simulink model "npc_controller"  (R2022a)
settings: Solver=FixedStepDiscrete  StartTime=0.0  StopTime=20  RelTol=1e-3  EnableMultiTasking=on
undefined symbols (not defined in the file): CAN_O_INT, CANA_BASE, Down, GPTRIP1SEL, GPTRIP2SEL, GPTRIP3SEL, Tsw, TZ1, TZ2, TZ3, Up
libraries: simulink x147, hdlsllib x90, c2802xlib x34, c2837xDlib x20, c280xlib x12, canmsglib x9, c2838xlib x8, idelinklib_common x3, c2806xlib x2, slpidlib x2, c28004xlib x2, c281xlib x2
(part 42 of 42)

== stateflow chart npc_controller/CONTROL/STATE-MACHINE/CPU_CONTROL_750_A2_precharge_pfc_ok2_OL SS1/detectUvpOvp/UVP ==
  (default) -> (junction 26)
  (junction 26) -> (junction 19) [order 1] : [Vpk2 < 536] %170Vacrms
  (junction 26) -> (junction 22) [order 2]
  (junction 19) -> (junction 23) : {
      | tfv_v_Uvp = 1; %set the UVP flag
      | }
  (junction 22) -> (junction 20) [order 1] : [Vpk2 > 568] %180Vacrms
  (junction 22) -> (junction 28) [order 2]
  (junction 20) -> (junction 18) : {
      | tfv_v_Uvp = 0;
      | }
  (junction 28) -> (junction 18)
  (junction 18) -> (junction 23)
  data: Vpk2 input single; tfv_v_Uvp output double

== stateflow chart npc_controller/CONTROL/STATE-MACHINE/CPU_CONTROL_750_A2_precharge_pfc_ok2_OL SS2 ==
  state configGrid(grid_config,   sinlgeph_config) [function] [commented out]
  state ClrCmpssTz [function] [commented out]
  state configFutEn [function]
  state disCmpssTz [function] [commented out]
  state configFutDis [function]
  state readCmpssOcp [function]
  state theta = updatePll3p(van, vbn, vcn) [function] [commented out]
  state calib_ok = updateCalib(cnt_calib, van, vbn, vcn, ia, ib, ic) [function]
  state disablePwm [function]
  state tfv_v_UvpOvp = detectUvpOvp(Vpk) [function]
  state phx_en = detectZCPhA(vxn) [function]
  state phx_en = detectZCPhB(vxn) [function]
  state phx_en = detectZCPhC(vxn) [function]
  state vx_seq = updateSequencePhA(vxn, ix) [function]
  state vx_seq = updateSequencePhB(vxn, ix) [function]
  state vx_seq = updateSequencePhC(vxn, ix) [function]
  (default) -> (junction 597)
  (junction 598) -> (junction 531) [order 1] : [calib_ok]
      | {tfv_v_UvpOvp = 0;//detectUvpOvp(Vpk);
      | readCmpssOcp();
      | }
  (junction 597) -> (junction 598) [order 1] : [start_cnt>1]%63333]//50cycles
  (junction 531) -> (junction 14)
  (junction 597) -> (junction 601) [order 2] : {
      | start_cnt++;
      | //disCmpssTz();
      | }
      | //exit
  (junction 598) -> (junction 539) [order 2] : {
      | calib_ok = updateCalib(cnt_calib, van, vbn, vcn, ia, ib, ic);
      | state = 0;
      | }
      | //exit
  (junction 14) -> (junction 542) [order 2]
  (junction 542) -> (junction 504) [order 2]
  (junction 504) -> (junction 506) [order 1] : [fut_en]
  (junction 14) -> (junction 128) [order 1] : /*fault latch*/
      | [tfv_va || tfv_vb || tfv_vc || tfv_iphasea || tfv_iphaseb || tfv_iphasec || tfv_vbulk || tfv_vmid /*|| tfv_vtop*/ || tfv_vaux || tz_ocp || tz_ovp || tz_cmpssocp || fault]
      | {
      | fault = true;
      | state = 1;
      | }
      | //turn OFF
  (junction 542) -> (junction 501) [order 1]
  (junction 504) -> (junction 512) [order 2]
  (junction 506) -> (junction 508) : {
      | configFutDis();
      | fut_en = false;
      | }
  (junction 508) -> (junction 512)
  (junction 501) -> (junction 490) : [fut_en_req]
  (junction 512) -> (junction 739)
  (junction 739) -> (junction 742) [commented out]
  (junction 490) -> (junction 492) [order 1] : [!fut_en]
  (junction 739) -> (junction 745) [order 2]
  (junction 742) -> (junction 735) [commented out] : [control_en]
  (junction 492) -> (junction 498) : {
      | configFutEn();
      | fut_en = true;
      | }
  (junction 490) -> (junction 494) [order 2]
  (junction 745) -> (junction 762) : {state = 7;}
      | //turn OFF
  (junction 739) -> (junction 734) [order 1] : [!tfv_v_UvpOvp]//check ac_ok at start
  (junction 494) -> (junction 498)
  (junction 735) -> (junction 734) [commented out]
  (junction 498) -> (junction 520) : {state = 2;}
  (junction 734) -> (junction 721)
  (junction 676) -> (junction 679) [order 1] : [control_en]
  (junction 721) -> (junction 712) [order 1] : [!pfc_en]
      | {state = 6;}
      | //turn OFF
      | //relay OFF
  (junction 721) -> (junction 778) [order 2]
  (junction 778) -> (junction 676) [order 1] : [delay_cnt > 100]//2666]
  (junction 679) -> (junction 678)
  (junction 778) -> (junction 780) [order 2] : {delay_cnt++;}
      | //exit
  (junction 676) -> (junction 346) [order 2]
  (junction 712) -> (junction 713)
  (junction 346) -> (junction 626) [order 1] : [(1.9797*2*Vpk-vbulk) < 50]
  (junction 346) -> (junction 558) [order 2]
  (junction 626) -> (junction 658) : {relay_ctrl = 1; //pre-charge relay ON
      | }
  (junction 658) -> (junction 678)
  (junction 678) -> (junction 622) [order 1] : [1]//relay_ctrl]
  (junction 558) -> (junction 658)
  (junction 622) -> (junction 624) [order 1] : [relay_cnt > 100]//3300] //PWM ON with 40ms delay
  (junction 624) -> (junction 754) [order 1] : [control_en]
  (junction 678) -> (junction 707) [order 2] : //exit
  (junction 622) -> (junction 623) [order 2] : {relay_cnt++;}
      | //exit
  (junction 624) -> (junction 699) [order 2]
  (junction 754) -> (junction 684)
  (junction 699) -> (junction 698) [order 1] : [vbulk > 2385] //540V
  (junction 699) -> (junction 692) [order 2]
  (junction 698) -> (junction 696) : {
      | control_en = 1; //PWM ON
      | ref = vbulk;
      | //enDigCmpMode();
      | //enCmpssTz();
      | }
  (junction 692) -> (junction 689) [order 1] : [vbulk < 2209] //500V
  (junction 692) -> (junction 691) [order 2]
  (junction 689) -> (junction 695) : {
      | control_en = false;
      | }
  (junction 684) -> (junction 114) [order 1] : [control_en]
  (junction 114) -> (junction 266) [order 1] : [vbulk > 5711] //840V
  (junction 696) -> (junction 684)
  (junction 691) -> (junction 695)
  (junction 695) -> (junction 696)
  (junction 684) -> (junction 665) [order 2] : //exit
  (junction 114) -> (junction 263) [order 2]
  (junction 266) -> (junction 273) : {
      | eoss = false;
      | burst_en = true;
      | }
  (junction 263) -> (junction 264) [order 1] : [vbulk < 3314] //750V
  (junction 263) -> (junction 267) [order 2]
  (junction 264) -> (junction 270) : {burst_en = false;}
  (junction 267) -> (junction 270)
  (junction 270) -> (junction 273)
  (junction 273) -> (junction 276) [order 1] : [burst_en]
  (junction 273) -> (junction 254) [order 2]
  (junction 276) -> (junction 327) : {
      | disablePwm();
      | va_seq = uint8(0); //forced zero
      | vb_seq = uint8(0);
      | vc_seq = uint8(0);
      | pha_en = false;
      | phb_en = false;
      | phc_en = false;
      | state = 5;
      | }
  (junction 254) -> (junction 256) [order 1] : [eoss]
      | //{tfv_v_UvpOvp = detectUvpOvp(Vpk)}
  (junction 256) -> (junction 648) [order 1] : [eoss_cnt > 6667]//5cycles delay after SS for PFC_OK
  (junction 254) -> (junction 97) [order 2]
  (junction 256) -> (junction 101) [order 2] : {
      | eoss_cnt++;
      | pfc_ok = 0;
      | }
  (junction 648) -> (junction 647) : {pfc_ok = 1;
      | /*eoss_cnt = 13100;*/}
  (junction 580) -> (junction 581) [commented out] : [(grid_config_req != grid_config) || (singleph_config_req != singleph_config)]
  (junction 97) -> (junction 93) [order 1] : [ref < 3314]%(single(883)-vbulk) > single(50)] //11V ripple
  (junction 580) -> (junction 583) [commented out]
  (junction 581) -> (junction 582) [commented out] : {
      | configGrid(grid_config,   singleph_config);
      | grid_config = grid_config_req;
      | singleph_config = singleph_config_req;
      | }
  (junction 97) -> (junction 110) [order 2]
  (junction 93) -> (junction 109) : {ref = ref + single(50);
      | eoss = false;}
  (junction 110) -> (junction 96) [commented out] : [(single(883)-vbulk) < single(-50)]
  (junction 110) -> (junction 94) : {ref = single(3314); //750V
      | eoss = true;}
  (junction 96) -> (junction 108) [commented out] : {ref = vbulk - single(1);
      | eoss = false;}
  (junction 101) -> (junction 647)
  (junction 647) -> (junction 352) [order 1] : [pha_en]
  (junction 109) -> (junction 101)
  (junction 582) -> (junction 583) [commented out]
  (junction 94) -> (junction 108)
  (junction 108) -> (junction 109)
  (junction 647) -> (junction 356) [order 2] : {
      | va_seq = uint8(0);
      | pha_en = detectZCPhA(van);
      | }
  (junction 352) -> (junction 354) : {va_seq = updateSequencePhA(van, ia);}
  (junction 583) -> (junction 133) [commented out]
  (junction 356) -> (junction 354)
  (junction 354) -> (junction 362) [order 1] : [phb_en]
  (junction 354) -> (junction 365) [order 2] : {
      | vb_seq = uint8(0);
      | phb_en = detectZCPhB(vbn);
      | }
  (junction 362) -> (junction 366) : {vb_seq = updateSequencePhB(vbn, ib);}
  (junction 365) -> (junction 366)
  (junction 366) -> (junction 367) [order 1] : [phc_en]
  (junction 366) -> (junction 370) [order 2] : {
      | vc_seq = uint8(0);
      | phc_en = detectZCPhC(vcn);
      | }
  (junction 367) -> (junction 372) : {vc_seq = updateSequencePhC(vcn, ic);}
  (junction 370) -> (junction 372)
  (junction 372) -> (junction 299) : {state = 4;}
  (junction 757) -> (junction 635) [order 1] : [!pfc_en || tfv_v_UvpOvp]
  (junction 635) -> (junction 299) [order 1] : [relayOff_cnt>2600] //40ms delay to turn-OFF pre-charge relay
      | {
      | relay_ctrl = 0; //pre-charge relay OFF
      | relayOff_cnt = 0;
      | relay_cnt = 0;
      | eoss_cnt = 0;
      | delay_cnt = 0;
      | }
  (junction 128) -> (junction 762) : //{calib_ok = false;} //calib_ok resets at fault or CAN command
  (junction 762) -> (junction 713)
  (junction 713) -> (junction 133)
  (junction 299) -> (junction 327)
  (junction 133) -> (junction 757) : {
      | disablePwm();
      | eoss = false;
      | //disDigCmpMode();
      | pha_en = false;
      | phb_en = false;
      | phc_en = false;
      | ref = vbulk;
      | %state = 3;
      | pfc_ok = 0;
      | control_en = false;
      | }
  (junction 635) -> (junction 637) [order 2] : {relayOff_cnt++;}
  (junction 632) -> (junction 299)
  (junction 327) -> (junction 533)
  (junction 757) -> (junction 759) [order 2]
  (junction 637) -> (junction 632)
  (junction 539) -> (junction 520)
  (junction 520) -> (junction 731)
  (junction 731) -> (junction 780)
  (junction 780) -> (junction 707)
  (junction 707) -> (junction 623)
  (junction 623) -> (junction 665)
  (junction 665) -> (junction 759)
  (junction 759) -> (junction 533)
  (junction 601) -> (junction 539)
  data: grid_config function_input double size=1; sinlgeph_config function_input double size=1; van function_input double size=1; vbn function_input double size=1; vcn function_input double size=1; theta function_output double size=1; calib_ok function_output; cnt_calib function_input uint16 size=1; van function_input single size=1; vbn function_input single size=1; vcn function_input single size=1; ia function_input single size=1; ib function_input single size=1; ic function_input single size=1; Vpk function_input; tfv_v_UvpOvp function_output; vxn function_input; phx_en function_output; vxn function_input; phx_en function_output; vxn function_input; phx_en function_output; vxn function_input; vx_seq function_output; ix function_input; vxn function_input; vx_seq function_output; ix function_input; vxn function_input; vx_seq function_output; ix function_input; state output uint16 =0; calib_ok output boolean =false; van input single; vbn input single; vcn input single; ia input single; ib input single; ic input single; tfv_vbulk data_store_memory; tfv_va data_store_memory; tfv_vmid data_store_memory; tfv_vb data_store_memory; tfv_vc data_store_memory; tfv_iphasea data_store_memory; tfv_iphaseb data_store_memory; tfv_iphasec data_store_memory; tfv_vtop data_store_memory; control_en output boolean =false; burst_en output boolean =false; eoss output boolean =false; ref output single =0; va_seq output uint8 =false; vb_seq output uint8 =false; vc_seq output uint8 =false; vbulk input single; fault local boolean =false; cnt_calib data_store_memory =0; theta data_store_memory =0; fut_en_req input uint8; fut_en local boolean =false; tfv_vaux data_store_memory; tz_ocp data_store_memory; tz_ovp data_store_memory; cnt_200ms local uint16 =0; pha_en output boolean =false; phb_en output boolean =false; phc_en output boolean =false; grid_config_req input uint8; singleph_config_req input uint8; grid_config local uint8 =0; singleph_config local uint8 =0; start_cnt local double; Vpk input single; relayOff_cnt local double; relay_cnt local double; pfc_ok output boolean; eoss_cnt local double; relay_ctrl output boolean; pfc_en input; tfv_v_UvpOvp output boolean; delay_cnt local double; tz_cmpssocp data_store_memory

== stateflow chart npc_controller/CONTROL/STATE-MACHINE/CPU_CONTROL_750_A2_precharge_pfc_ok2_OL SS2/detectUvpOvp/OVP ==
  (default) -> (junction 5)
  (junction 5) -> (junction 4) [order 1] : [Vpk1 > 773] %245Vacrms
  (junction 5) -> (junction 7) [order 2]
  (junction 4) -> (junction 6) : {
      | tfv_v_Ovp = 1; %set the OVP flag
      | }
  (junction 7) -> (junction 2) [order 1] : [Vpk1 < 741] %235Vacrms
  (junction 7) -> (junction 1) [order 2]
  (junction 2) -> (junction 3) : {
      | tfv_v_Ovp = 0;
      | }
  (junction 1) -> (junction 3)
  (junction 3) -> (junction 6)
  data: Vpk1 input single; tfv_v_Ovp output double

== stateflow chart npc_controller/CONTROL/STATE-MACHINE/CPU_CONTROL_750_A2_precharge_pfc_ok2_OL SS2/detectUvpOvp/UVP ==
  (default) -> (junction 26)
  (junction 26) -> (junction 19) [order 1] : [Vpk2 < 536] %170Vacrms
  (junction 26) -> (junction 22) [order 2]
  (junction 19) -> (junction 23) : {
      | tfv_v_Uvp = 1; %set the UVP flag
      | }
  (junction 22) -> (junction 20) [order 1] : [Vpk2 > 568] %180Vacrms
  (junction 22) -> (junction 28) [order 2]
  (junction 20) -> (junction 18) : {
      | tfv_v_Uvp = 0;
      | }
  (junction 28) -> (junction 18)
  (junction 18) -> (junction 23)
  data: Vpk2 input single; tfv_v_Uvp output double

== stateflow chart npc_controller/CONTROL/SVPWM/SVPWM_with_bal ==
  state [Tx,Ty,Tz] = calcDwellingTimes(Tsw,vref_fict_mag_alpha,vref_fict_mag_beta,vx_fict_mag_alpha,vx_fict_mag_beta,vy_fict_mag_alpha,vy_fict_mag_beta) [function]
  state [r_seq, s_seq, t_seq]=detSeq(subsector) [function]
  state [r_seq, s_seq, t_seq]=detSeqFixedSmallVector(subsector) [function] [commented out]
  state [cmp_r, cmp_s, cmp_t] = calcCmp(r_seq, s_seq, t_seq, Tx, Ty, Tz) [function] [commented out]
  state [cmp_r, cmp_s, cmp_t] = calcCmpWithBal(r_seq, s_seq, t_seq, Tx, Ty, Tz) [function]
  (default) -> (junction 4)
  (junction 4) -> (junction 6) [order 1] : [vref_mag_alpha >= 0]
  (junction 6) -> (junction 12) [order 1] : [vref_mag_beta >= 0]
  (junction 12) -> (junction 14) [order 1] : [vref_mag_beta > (vref_mag_alpha*tan(3.14/6))]
  (junction 4) -> (junction 8) [order 2]
  (junction 6) -> (junction 23) [order 2]
  (junction 12) -> (junction 19) [order 2] : {main_sector = 1;}
  (junction 14) -> (junction 16) : {main_sector = 2;}
  (junction 19) -> (junction 16)
  (junction 16) -> (junction 54)
  (junction 23) -> (junction 25) [order 1] : [vref_mag_beta < (-vref_mag_alpha*tan(3.14/6))]
  (junction 23) -> (junction 29) [order 2] : {main_sector = 1;}
  (junction 25) -> (junction 27) : {main_sector = 6;}
  (junction 29) -> (junction 27)
  (junction 27) -> (junction 54)
  (junction 54) -> (junction 52)
  (junction 32) -> (junction 39) [order 1] : [vref_mag_beta > (abs(vref_mag_alpha)*tan(3.14/6))]
  (junction 8) -> (junction 32) [order 1] : [vref_mag_beta >= 0]
  (junction 39) -> (junction 40) : {main_sector = 3;}
  (junction 8) -> (junction 35) [order 2]
  (junction 32) -> (junction 41) [order 2] : {main_sector = 4;}
  (junction 41) -> (junction 40)
  (junction 40) -> (junction 52)
  (junction 52) -> (junction 21)
  (junction 35) -> (junction 44) [order 1] : [vref_mag_beta < (vref_mag_alpha*tan(3.14/6))]
  (junction 35) -> (junction 46) [order 2] : {main_sector = 4;}
  (junction 44) -> (junction 48) : {main_sector = 5;}
  (junction 46) -> (junction 48)
  (junction 48) -> (junction 21)
  (junction 21) -> (junction 63)
  (junction 63) -> (junction 64) [order 1] : [main_sector == 1]
  (junction 63) -> (junction 65) [order 2]
  (junction 64) -> (junction 86) : {
      | mapv_mag_alpha = 0.3333;
      | mapv_mag_beta = 0;
      | }
  (junction 65) -> (junction 69) [order 1] : [main_sector == 2]
  (junction 65) -> (junction 67) [order 2]
  (junction 69) -> (junction 72) : {
      | mapv_mag_alpha = 0.1667;
      | mapv_mag_beta = 0.2887;
      | }
  (junction 67) -> (junction 68) [order 1] : [main_sector == 3]
  (junction 67) -> (junction 58) [order 2]
  (junction 68) -> (junction 95) : {
      | mapv_mag_alpha = -0.1667;
      | mapv_mag_beta = 0.2887;
      | }
  (junction 58) -> (junction 66) [order 1] : [main_sector == 4]
  (junction 58) -> (junction 59) [order 2]
  (junction 66) -> (junction 93) : {
      | mapv_mag_alpha = -0.3333;
      | mapv_mag_beta = 0;
      | }
  (junction 59) -> (junction 60) [order 1] : [main_sector == 5]
  (junction 59) -> (junction 61) [order 2]
  (junction 60) -> (junction 91) : {
      | mapv_mag_alpha = -0.1667;
      | mapv_mag_beta = -0.2887;
      | }
  (junction 61) -> (junction 62) [order 1] : [main_sector == 6]
  (junction 61) -> (junction 83) [order 2]
  (junction 62) -> (junction 90) : {
      | mapv_mag_alpha = 0.1667;
      | mapv_mag_beta = -0.2887;
      | }
  (junction 83) -> (junction 90)
  (junction 90) -> (junction 91)
  (junction 91) -> (junction 93)
  (junction 93) -> (junction 95)
  (junction 95) -> (junction 72)
  (junction 72) -> (junction 86)
  (junction 86) -> (junction 145) : {
      | vref_fict_mag_alpha = vref_mag_alpha - mapv_mag_alpha;
      | vref_fict_mag_beta = vref_mag_beta - mapv_mag_beta;
      | }
  (junction 145) -> (junction 146) [order 1] : [vref_fict_mag_alpha >= 0]
  (junction 146) -> (junction 147) [order 1] : [vref_fict_mag_beta >= 0]
  (junction 147) -> (junction 148) [order 1] : [vref_fict_mag_beta > (vref_fict_mag_alpha*tan(3.14/3))]
  (junction 145) -> (junction 158) [order 2]
  (junction 146) -> (junction 149) [order 2]
  (junction 147) -> (junction 150) [order 2] : {subsector = 1;}
  (junction 148) -> (junction 151) : {subsector = 2;}
  (junction 150) -> (junction 151)
  (junction 151) -> (junction 159)
  (junction 149) -> (junction 152) [order 1] : [vref_fict_mag_beta < (-vref_fict_mag_alpha*tan(3.14/3))]
  (junction 149) -> (junction 153) [order 2] : {subsector = 6;}
  (junction 152) -> (junction 154) : {subsector = 5;}
  (junction 153) -> (junction 154)
  (junction 154) -> (junction 159)
  (junction 159) -> (junction 109)
  (junction 156) -> (junction 155) [order 1] : [vref_fict_mag_beta > (abs(vref_fict_mag_alpha)*tan(3.14/3))]
  (junction 158) -> (junction 156) [order 1] : [vref_fict_mag_beta >= 0]
  (junction 155) -> (junction 122) : {subsector = 2;}
  (junction 158) -> (junction 126) [order 2]
  (junction 156) -> (junction 157) [order 2] : {subsector = 3;}
  (junction 157) -> (junction 122)
  (junction 122) -> (junction 109)
  (junction 109) -> (junction 128)
  (junction 126) -> (junction 127) [order 1] : [vref_fict_mag_beta < (vref_fict_mag_alpha*tan(3.14/3))]
  (junction 126) -> (junction 129) [order 2] : {subsector = 4;}
  (junction 127) -> (junction 130) : {subsector = 5;}
  (junction 129) -> (junction 130)
  (junction 130) -> (junction 128)
  (junction 128) -> (junction 182)
  (junction 182) -> (junction 162) [order 1] : [subsector == 1]
  (junction 182) -> (junction 163) [order 2]
  (junction 162) -> (junction 179) : {
      | vx_fict_mag_alpha = 0.3333;
      | vx_fict_mag_beta = 0;
      | vy_fict_mag_alpha = 0.1667;
      | vy_fict_mag_beta = 0.2887;
      | }
  (junction 163) -> (junction 164) [order 1] : [subsector == 2]
  (junction 163) -> (junction 177) [order 2]
  (junction 164) -> (junction 178) : {
      | vx_fict_mag_alpha = 0.1667;
      | vx_fict_mag_beta = 0.2887;
      | vy_fict_mag_alpha = -0.1667;
      | vy_fict_mag_beta = 0.2887;
      | }
  (junction 177) -> (junction 167) [order 1] : [subsector == 3]
  (junction 177) -> (junction 174) [order 2]
  (junction 167) -> (junction 172) : {
      | vx_fict_mag_alpha = -0.1667;
      | vx_fict_mag_beta = 0.2887;
      | vy_fict_mag_alpha = -0.3333;
      | vy_fict_mag_beta = 0;
      | }
  (junction 174) -> (junction 173) [order 1] : [subsector == 4]
  (junction 174) -> (junction 175) [order 2]
  (junction 173) -> (junction 170) : {
      | vx_fict_mag_alpha = -0.3333;
      | vx_fict_mag_beta = 0;
      | vy_fict_mag_alpha = -0.1667;
      | vy_fict_mag_beta = -0.2887;
      | }
  (junction 175) -> (junction 165) [order 1] : [subsector == 5]
  (junction 175) -> (junction 166) [order 2]
  (junction 165) -> (junction 176) : {
      | vx_fict_mag_alpha = -0.1667;
      | vx_fict_mag_beta = -0.2887;
      | vy_fict_mag_alpha = 0.1667;
      | vy_fict_mag_beta = -0.2887;
      | }
  (junction 166) -> (junction 171) [order 1] : [subsector == 6]
  (junction 166) -> (junction 168) [order 2]
  (junction 171) -> (junction 169) : {
      | vx_fict_mag_alpha = 0.1667;
      | vx_fict_mag_beta = -0.2887;
      | vy_fict_mag_alpha = 0.3333;
      | vy_fict_mag_beta = 0;
      | }
  (junction 168) -> (junction 169)
  (junction 169) -> (junction 176)
  (junction 176) -> (junction 170)
  (junction 170) -> (junction 172)
  (junction 172) -> (junction 178)
  (junction 178) -> (junction 179)
  (junction 179) -> (junction 232) : {
      | [Tx, Ty, Tz] = calcDwellingTimes(Tsw, vref_fict_mag_alpha, vref_fict_mag_beta, vx_fict_mag_alpha, vx_fict_mag_beta, vy_fict_mag_alpha, vy_fict_mag_beta);
      | }
  (junction 232) -> (junction 247) : {
      | [r_seq, s_seq, t_seq]=detSeq(subsector);
      | }
  (junction 247) -> (junction 334) : {[cmp_r, cmp_s, cmp_t] = calcCmpWithBal(r_seq, s_seq, t_seq, Tx, Ty, Tz);}
  (junction 334) -> (junction 262)
  (junction 262) -> (junction 253) [order 1] : [main_sector == 1]
  (junction 262) -> (junction 258) [order 2]
  (junction 253) -> (junction 283) : {
      | r_p = cmp_r+midpt_bal_coef;
      | r_n = 0;
      | s_p = 0;
      | s_n = -cmp_s+1;
      | t_p = 0;
      | t_n = -cmp_t+1;
      | }
  (junction 258) -> (junction 254) [order 1] : [main_sector == 2]
  (junction 258) -> (junction 255) [order 2]
  (junction 254) -> (junction 276) : {
      | r_p = cmp_r+midpt_bal_coef;
      | r_n = 0;
      | s_p = cmp_s+midpt_bal_coef;
      | s_n = 0;
      | t_p = 0;
      | t_n = -cmp_t+1;
      | }
  (junction 255) -> (junction 250) [order 1] : [main_sector == 3]
  (junction 255) -> (junction 256) [order 2]
  (junction 250) -> (junction 266) : {
      | r_p = 0;
      | r_n = -cmp_r+1;
      | s_p = cmp_s+midpt_bal_coef;
      | s_n = 0;
      | t_p = 0;
      | t_n = -cmp_t+1;
      | }
  (junction 256) -> (junction 257) [order 1] : [main_sector == 4]
  (junction 256) -> (junction 261) [order 2]
  (junction 257) -> (junction 265) : {
      | r_p = 0;
      | r_n = -cmp_r+1;
      | s_p = cmp_s+midpt_bal_coef;
      | s_n = 0;
      | t_p = cmp_t+midpt_bal_coef;
      | t_n = 0;
      | }
  (junction 261) -> (junction 251) [order 1] : [main_sector == 5]
  (junction 261) -> (junction 259) [order 2]
  (junction 251) -> (junction 264) : {
      | r_p = 0;
      | r_n = -cmp_r+1;
      | s_p = 0;
      | s_n = -cmp_s+1;
      | t_p = cmp_t+midpt_bal_coef;
      | t_n = 0;
      | }
  (junction 259) -> (junction 260) [order 1] : [main_sector == 6]
  (junction 259) -> (junction 252) [order 2]
  (junction 260) -> (junction 263) : {
      | r_p = cmp_r+midpt_bal_coef;
      | r_n = 0;
      | s_p = 0;
      | s_n = -cmp_s+1;
      | t_p = cmp_t+midpt_bal_coef;
      | t_n = 0;
      | }
  (junction 252) -> (junction 263)
  (junction 263) -> (junction 264)
  (junction 264) -> (junction 265)
  (junction 265) -> (junction 266)
  (junction 266) -> (junction 276)
  (junction 276) -> (junction 283)
  (junction 283) -> (junction 316) : {
      | debug_a = main_sector;
      | debug_b = subsector;
      | debug_c = cmp_r;
      | }
  data: Tsw function_input double size=1; vref_fict_mag_alpha function_input double size=1; vref_fict_mag_beta function_input double size=1; Tx function_output; Ty function_output; Tz function_output; vx_fict_mag_alpha function_input double size=1; vx_fict_mag_beta function_input double size=1; vy_fict_mag_alpha function_input double size=1; vy_fict_mag_beta function_input double size=1; subsector function_input double size=1; r_seq function_output; s_seq function_output; t_seq function_output; subsector function_input double size=1; r_seq function_output double size=1; s_seq function_output double size=1; t_seq function_output double size=1; r_seq function_input double size=1; cmp_r function_output double size=1; cmp_s function_output double size=1; cmp_t function_output double size=1; s_seq function_input double size=1; t_seq function_input double size=1; Tx function_input double size=1; Ty function_input double size=1; Tz function_input double size=1; r_seq function_input double size=4; cmp_r function_output; cmp_s function_output; cmp_t function_output; s_seq function_input double size=4; t_seq function_input double size=4; Tx function_input double size=1; Ty function_input double size=1; Tz function_input double size=1; r_p output double; r_n output double; vref_mag_alpha input double; vref_mag_beta input double; mapv_mag_alpha local double; mapv_mag_beta local double; vref_fict_mag_alpha local double; vref_fict_mag_beta local double; subsector local double; main_sector local double; vx_fict_mag_alpha local double; vx_fict_mag_beta local double; vy_fict_mag_alpha local double; vy_fict_mag_beta local double; midpt_bal_coef input double; Tx local double; Ty local double; Tz local double; s_p output double; s_n output double; t_p output double; t_n output double; cmp_r local double; cmp_s local double; cmp_t local double; r_seq local double size=4; s_seq local double size=4; t_seq local double size=4; debug_a output double; debug_b output double; debug_c output double; Tsw input double

== stateflow chart npc_controller/CONTROL/SVPWM/SVPWM2 ==
  state [Tx,Ty,Tz] = calcDwellingTimes(Tsw,vref_fict_mag_alpha,vref_fict_mag_beta,vx_fict_mag_alpha,vx_fict_mag_beta,vy_fict_mag_alpha,vy_fict_mag_beta) [function]
  state [r_seq, s_seq, t_seq]=detSeq(subsector) [function]
  state [cmp_r,cmp_s,cmp_t] = calcCmpBal(r_seq,s_seq,t_seq,Tx,Ty,Tz,vbal_coef) [function]
  (default) -> (junction 4)
  (junction 4) -> (junction 6) [order 1] : [vref_mag_alpha >= 0]
  (junction 6) -> (junction 12) [order 1] : [vref_mag_beta >= 0]
  (junction 12) -> (junction 14) [order 1] : [vref_mag_beta > (vref_mag_alpha*0.5774)]
  (junction 4) -> (junction 8) [order 2]
  (junction 6) -> (junction 23) [order 2]
  (junction 12) -> (junction 19) [order 2] : {main_sector = 1;}
  (junction 14) -> (junction 16) : {main_sector = 2;}
  (junction 19) -> (junction 16)
  (junction 16) -> (junction 54)
  (junction 23) -> (junction 25) [order 1] : [vref_mag_beta < (-vref_mag_alpha*0.5774)]
  (junction 23) -> (junction 29) [order 2] : {main_sector = 1;}
  (junction 25) -> (junction 27) : {main_sector = 6;}
  (junction 29) -> (junction 27)
  (junction 27) -> (junction 54)
  (junction 54) -> (junction 52)
  (junction 32) -> (junction 39) [order 1] : [vref_mag_beta > (abs(vref_mag_alpha)*0.5774)]
  (junction 8) -> (junction 32) [order 1] : [vref_mag_beta >= 0]
  (junction 39) -> (junction 40) : {main_sector = 3;}
  (junction 8) -> (junction 35) [order 2]
  (junction 32) -> (junction 41) [order 2] : {main_sector = 4;}
  (junction 41) -> (junction 40)
  (junction 40) -> (junction 52)
  (junction 52) -> (junction 378)
  (junction 35) -> (junction 44) [order 1] : [vref_mag_beta < (vref_mag_alpha*0.5774)]
  (junction 35) -> (junction 46) [order 2] : {main_sector = 4;}
  (junction 44) -> (junction 48) : {main_sector = 5;}
  (junction 46) -> (junction 48)
  (junction 48) -> (junction 378)
  (junction 378) -> (junction 379)
  (junction 379) -> (junction 64) [order 1] : [main_sector == 1]
  (junction 379) -> (junction 65) [order 2]
  (junction 64) -> (junction 86) : {
      | mapv_mag_alpha = 0.3333;
      | mapv_mag_beta = 0;
      | }
  (junction 65) -> (junction 69) [order 1] : [main_sector == 2]
  (junction 65) -> (junction 67) [order 2]
  (junction 69) -> (junction 72) : {
      | mapv_mag_alpha = 0.1667;
      | mapv_mag_beta = 0.2887;
      | }
  (junction 67) -> (junction 68) [order 1] : [main_sector == 3]
  (junction 67) -> (junction 58) [order 2]
  (junction 68) -> (junction 95) : {
      | mapv_mag_alpha = -0.1667;
      | mapv_mag_beta = 0.2887;
      | }
  (junction 58) -> (junction 66) [order 1] : [main_sector == 4]
  (junction 58) -> (junction 59) [order 2]
  (junction 66) -> (junction 93) : {
      | mapv_mag_alpha = -0.3333;
      | mapv_mag_beta = 0;
      | }
  (junction 59) -> (junction 60) [order 1] : [main_sector == 5]
  (junction 59) -> (junction 376) [order 2] : {
      | mapv_mag_alpha = 0.1667;
      | mapv_mag_beta = -0.2887;
      | }
  (junction 60) -> (junction 91) : {
      | mapv_mag_alpha = -0.1667;
      | mapv_mag_beta = -0.2887;
      | }
  (junction 376) -> (junction 91)
  (junction 91) -> (junction 93)
  (junction 93) -> (junction 95)
  (junction 95) -> (junction 72)
  (junction 72) -> (junction 86)
  (junction 86) -> (junction 145) : {
      | vref_fict_mag_alpha = vref_mag_alpha - mapv_mag_alpha;
      | vref_fict_mag_beta = vref_mag_beta - mapv_mag_beta;
      | }
  (junction 145) -> (junction 146) [order 1] : [vref_fict_mag_alpha >= 0]
  (junction 146) -> (junction 147) [order 1] : [vref_fict_mag_beta >= 0]
  (junction 147) -> (junction 148) [order 1] : [vref_fict_mag_beta > (vref_fict_mag_alpha*1.7299)]
  (junction 145) -> (junction 158) [order 2]
  (junction 146) -> (junction 149) [order 2]
  (junction 147) -> (junction 150) [order 2] : {subsector = 1;}
  (junction 148) -> (junction 151) : {subsector = 2;}
  (junction 150) -> (junction 151)
  (junction 151) -> (junction 159)
  (junction 149) -> (junction 152) [order 1] : [vref_fict_mag_beta < (-vref_fict_mag_alpha*1.7299)]
  (junction 149) -> (junction 153) [order 2] : {subsector = 6;}
  (junction 152) -> (junction 154) : {subsector = 5;}
  (junction 153) -> (junction 154)
  (junction 154) -> (junction 159)
  (junction 159) -> (junction 109)
  (junction 156) -> (junction 155) [order 1] : [vref_fict_mag_beta > (abs(vref_fict_mag_alpha)*1.7299)]
  (junction 158) -> (junction 156) [order 1] : [vref_fict_mag_beta >= 0]
  (junction 155) -> (junction 122) : {subsector = 2;}
  (junction 158) -> (junction 126) [order 2]
  (junction 156) -> (junction 157) [order 2] : {subsector = 3;}
  (junction 157) -> (junction 122)
  (junction 122) -> (junction 109)
  (junction 109) -> (junction 128)
  (junction 126) -> (junction 127) [order 1] : [vref_fict_mag_beta < (vref_fict_mag_alpha*1.7299)]
  (junction 126) -> (junction 129) [order 2] : {subsector = 4;}
  (junction 127) -> (junction 130) : {subsector = 5;}
  (junction 129) -> (junction 130)
  (junction 130) -> (junction 128)
  (junction 128) -> (junction 182)
  (junction 182) -> (junction 162) [order 1] : [subsector == 1]
  (junction 182) -> (junction 163) [order 2]
  (junction 162) -> (junction 179) : {
      | vx_fict_mag_alpha = 0.3333;
      | vx_fict_mag_beta = 0;
      | vy_fict_mag_alpha = 0.1667;
      | vy_fict_mag_beta = 0.2887;
      | }
  (junction 163) -> (junction 164) [order 1] : [subsector == 2]
  (junction 163) -> (junction 177) [order 2]
  (junction 164) -> (junction 178) : {
      | vx_fict_mag_alpha = 0.1667;
      | vx_fict_mag_beta = 0.2887;
      | vy_fict_mag_alpha = -0.1667;
      | vy_fict_mag_beta = 0.2887;
      | }
  (junction 177) -> (junction 167) [order 1] : [subsector == 3]
  (junction 177) -> (junction 174) [order 2]
  (junction 167) -> (junction 172) : {
      | vx_fict_mag_alpha = -0.1667;
      | vx_fict_mag_beta = 0.2887;
      | vy_fict_mag_alpha = -0.3333;
      | vy_fict_mag_beta = 0;
      | }
  (junction 174) -> (junction 173) [order 1] : [subsector == 4]
  (junction 174) -> (junction 175) [order 2]
  (junction 173) -> (junction 170) : {
      | vx_fict_mag_alpha = -0.3333;
      | vx_fict_mag_beta = 0;
      | vy_fict_mag_alpha = -0.1667;
      | vy_fict_mag_beta = -0.2887;
      | }
  (junction 175) -> (junction 165) [order 1] : [subsector == 5]
  (junction 175) -> (junction 381) [order 2] : {
      | vx_fict_mag_alpha = 0.1667;
      | vx_fict_mag_beta = -0.2887;
      | vy_fict_mag_alpha = 0.3333;
      | vy_fict_mag_beta = 0;
      | }
  (junction 165) -> (junction 176) : {
      | vx_fict_mag_alpha = -0.1667;
      | vx_fict_mag_beta = -0.2887;
      | vy_fict_mag_alpha = 0.1667;
      | vy_fict_mag_beta = -0.2887;
      | }
  (junction 381) -> (junction 176)
  (junction 176) -> (junction 170)
  (junction 170) -> (junction 172)
  (junction 172) -> (junction 178)
  (junction 178) -> (junction 179)
  (junction 179) -> (junction 232) : {
      | [Tx, Ty, Tz] = calcDwellingTimes(Tsw, vref_fict_mag_alpha, vref_fict_mag_beta, vx_fict_mag_alpha, vx_fict_mag_beta, vy_fict_mag_alpha, vy_fict_mag_beta);
      | }
  (junction 232) -> (junction 247) : {
      | [r_seq, s_seq, t_seq]=detSeq(subsector);
      | }
  (junction 247) -> (junction 262) : {[cmp_r, cmp_s, cmp_t] = calcCmpBal(r_seq, s_seq, t_seq, Tx, Ty, Tz, vbal_coef);}
  (junction 262) -> (junction 253) [order 1] : [main_sector == 1]
  (junction 262) -> (junction 258) [order 2]
  (junction 253) -> (junction 283) : {
      | r_p = cmp_r;
      | r_n = 0;
      | s_p = 0;
      | s_n = -cmp_s+1;
      | t_p = 0;
      | t_n = -cmp_t+1;
      | }
  (junction 258) -> (junction 254) [order 1] : [main_sector == 2]
  (junction 258) -> (junction 255) [order 2]
  (junction 254) -> (junction 276) : {
      | r_p = cmp_r
      | r_n = 0;
      | s_p = cmp_s;
      | s_n = 0;
      | t_p = 0;
      | t_n = -cmp_t+1;
      | }
  (junction 255) -> (junction 250) [order 1] : [main_sector == 3]
  (junction 255) -> (junction 256) [order 2]
  (junction 250) -> (junction 266) : {
      | r_p = 0;
      | r_n = -cmp_r+1;
      | s_p = cmp_s;
      | s_n = 0;
      | t_p = 0;
      | t_n = -cmp_t+1;
      | }
  (junction 256) -> (junction 257) [order 1] : [main_sector == 4]
  (junction 256) -> (junction 261) [order 2]
  (junction 257) -> (junction 265) : {
      | r_p = 0;
      | r_n = -cmp_r+1;
      | s_p = cmp_s;
      | s_n = 0;
      | t_p = cmp_t;
      | t_n = 0;
      | }
  (junction 261) -> (junction 251) [order 1] : [main_sector == 5]
  (junction 261) -> (junction 383) [order 2] : {
      | r_p = cmp_r;
      | r_n = 0;
      | s_p = 0;
      | s_n = -cmp_s+1;
      | t_p = cmp_t;
      | t_n = 0;
      | }
  (junction 251) -> (junction 264) : {
      | r_p = 0;
      | r_n = -cmp_r+1;
      | s_p = 0;
      | s_n = -cmp_s+1;
      | t_p = cmp_t;
      | t_n = 0;
      | }
  (junction 383) -> (junction 264)
  (junction 264) -> (junction 265)
  (junction 265) -> (junction 266)
  (junction 266) -> (junction 276)
  (junction 276) -> (junction 283)
  (junction 283) -> (junction 313) : {
      | debug_a = vref_mag_alpha;
      | debug_b = vref_mag_beta;
      | debug_c = main_sector;
      | debug_d = subsector;
      | debug_e = vref_fict_mag_alpha;
      | debug_f = vref_fict_mag_beta;
      | }
  data: Tsw function_input double size=1; vref_fict_mag_alpha function_input double size=1; vref_fict_mag_beta function_input double size=1; Tx function_output; Ty function_output; Tz function_output; vx_fict_mag_alpha function_input double size=1; vx_fict_mag_beta function_input double size=1; vy_fict_mag_alpha function_input double size=1; vy_fict_mag_beta function_input double size=1; subsector function_input double size=1; r_seq function_output; s_seq function_output; t_seq function_output; r_seq function_input double size=4; cmp_r function_output; cmp_s function_output; cmp_t function_output; s_seq function_input double size=4; t_seq function_input double size=4; Tx function_input double size=1; Ty function_input double size=1; Tz function_input double size=1; vbal_coef function_input; r_p output double; r_n output double; vref_mag_alpha input double; vref_mag_beta input double; mapv_mag_alpha local double; mapv_mag_beta local double; vref_fict_mag_alpha local double; vref_fict_mag_beta local double; subsector local double; main_sector local double; vx_fict_mag_alpha local double; vx_fict_mag_beta local double; vy_fict_mag_alpha local double; vy_fict_mag_beta local double; vbal_coef input double; Tx local double; Ty local double; Tz local double; s_p output double; s_n output double; t_p output double; t_n output double; cmp_r local double; cmp_s local double; cmp_t local double; r_seq local double size=4; s_seq local double size=4; t_seq local double size=4; debug_a output double; debug_b output double; debug_c output double; debug_d output double; debug_e output double; debug_f output double; pi local double =3.1415926535; Tsw input double

== stateflow chart npc_controller/IDLE_AND_TIMER/codegen/IDLE/idle_task1/hkeep/tfv/hkeep1 ==
  state HKEEP
    du:
    tfv_va = tfvVa(uint16(adc_va), uint16(2940), uint16(3), uint16(1), uint16(3)); //400Vac,pk
    tfv_vb = tfvVb(uint16(adc_vb), uint16(2940), uint16(3), uint16(1), uint16(3)); //400Vac,pk
    tfv_vc = tfvVc(uint16(adc_vc), uint16(2940), uint16(3), uint16(1), uint16(3)); //400Vac,pk
    //tfv_iphasea = tfvIphaseA(uint16(adc_iphasea), uint16(2100), uint16(1), uint16(1), uint16(3)); //2A
    //tfv_iphaseb = tfvIphaseB(uint16(adc_iphaseb), uint16(2100), uint16(1), uint16(1), uint16(3)); //2A
    //tfv_iphasec = tfvIphaseC(uint16(adc_iphasec), uint16(2100), uint16(1), uint16(1), uint16(3)); //2A
    tfv_vbulk = tfvVbulk(uint16(adc_vbulk), uint16(3821), uint16(3), uint16(1), uint16(3)); //850V
    tfv_vmid = tfvVmid(uint16(adc_vmid), uint16(3443), uint16(3), uint16(1), uint16(3)); //430V
    tfv_vaux = tfvVaux(uint16(adc_vaux), uint16(3722), uint16(3), uint16(1), uint16(3)); //3V
    state tfv_va = tfvVa(input, assert_lim, assert_vld, deassert_lim, deassert_vld) [function]
    state tfv_vb = tfvVb(input, assert_lim, assert_vld, deassert_lim, deassert_vld) [function]
    state tfv_vc = tfvVc(input, assert_lim, assert_vld, deassert_lim, deassert_vld) [function]
    state tfv_iphasaea = tfvIphaseA(input, assert_lim, assert_vld, deassert_lim, deassert_vld) [function] [commented out]
    state tfv_iphaseb = tfvIphaseB(input, assert_lim, assert_vld, deassert_lim, deassert_vld) [function] [commented out]
    state tfv_iphasec = tfvIphaseC(input, assert_lim, assert_vld, deassert_lim, deassert_vld) [function] [commented out]
    state tfv_vbulk = tfvVbulk(input, assert_lim, assert_vld, deassert_lim, deassert_vld) [function]
    state tfv_vmid = tfvVmid(input, assert_lim, assert_vld, deassert_lim, deassert_vld) [function]
    state tfv_vaux = tfvVaux(input, assert_lim, assert_vld, deassert_lim, deassert_vld) [function]
  (default) -> HKEEP
  data: tfv_va function_output boolean; input function_input uint16 size=1; assert_lim function_input uint16 size=1; assert_vld function_input uint16 size=1; deassert_lim function_input uint16 size=1; deassert_vld function_input uint16 size=1; tfv_vb function_output boolean; input function_input uint16 size=1; assert_lim function_input uint16 size=1; assert_vld function_input uint16 size=1; deassert_lim function_input uint16 size=1; deassert_vld function_input uint16 size=1; tfv_vc function_output boolean; input function_input uint16 size=1; assert_lim function_input uint16 size=1; assert_vld function_input uint16 size=1; deassert_lim function_input uint16 size=1; deassert_vld function_input uint16 size=1; tfv_iphasaea function_output double size=1; input function_input double size=1; assert_lim function_input double size=1; assert_vld function_input double size=1; deassert_lim function_input double size=1; deassert_vld function_input double size=1; tfv_iphaseb function_output double size=1; input function_input double size=1; assert_lim function_input double size=1; assert_vld function_input double size=1; deassert_lim function_input double size=1; deassert_vld function_input double size=1; tfv_iphasec function_output double size=1; input function_input double size=1; assert_lim function_input double size=1; assert_vld function_input double size=1; deassert_lim function_input double size=1; deassert_vld function_input double size=1; tfv_vbulk function_output boolean; input function_input uint16 size=1; assert_lim function_input uint16 size=1; assert_vld function_input uint16 size=1; deassert_lim function_input uint16 size=1; deassert_vld function_input uint16 size=1; tfv_vmid function_output boolean; input function_input uint16 size=1; assert_lim function_input uint16 size=1; assert_vld function_input uint16 size=1; deassert_lim function_input uint16 size=1; deassert_vld function_input uint16 size=1; tfv_vaux function_output boolean; input function_input uint16 size=1; assert_lim function_input uint16 size=1; assert_vld function_input uint16 size=1; deassert_lim function_input uint16 size=1; deassert_vld function_input uint16 size=1; tfv_vout local double; tfv_vbulk data_store_memory; tfv_vmid data_store_memory; tfv_va data_store_memory; tfv_vb data_store_memory; tfv_vc data_store_memory; tfv_iphasec data_store_memory; tfv_iphaseb data_store_memory; tfv_iphasea data_store_memory; adc_vmid data_store_memory; adc_vbulk data_store_memory; adc_va data_store_memory; adc_vb data_store_memory; adc_vc data_store_memory; adc_iphasea data_store_memory; adc_iphasec data_store_memory; adc_iphaseb data_store_memory; tfv_vtop data_store_memory; adc_vtop data_store_memory; tfv_vaux data_store_memory; adc_vaux data_store_memory

== stateflow chart npc_controller/CONTROL/STATE-MACHINE/CPU_CONTROL_400 ==
  state configGrid(grid_config,   sinlgeph_config) [function] [commented out]
  state enDigCmpMode [function]
  state configFutEn [function]
  state disDigCmpMode [function]
  state configFutDis [function]
  state theta = updatePll3p(van, vbn, vcn) [function] [commented out]
  state calib_ok = updateCalib(cnt_calib, van, vbn, vcn, ia, ib, ic) [function]
  state disablePwm [function]
  state phx_en = detectZCPhA(vxn) [function]
  state phx_en = detectZCPhB(vxn) [function]
  state phx_en = detectZCPhC(vxn) [function]
  state vx_seq = updateSequencePhA(vxn, ix) [function]
  state vx_seq = updateSequencePhB(vxn, ix) [function]
  state vx_seq = updateSequencePhC(vxn, ix) [function]
  (default) -> (junction 437) : //{calib_ok = true;}
  (junction 437) -> (junction 531) [order 1] : [calib_ok]
  (junction 437) -> (junction 539) [order 2] : {
      | calib_ok = updateCalib(cnt_calib, van, vbn, vcn, ia, ib, ic);
      | state = 0;
      | }
  (junction 531) -> (junction 14)
  (junction 14) -> (junction 542) [order 2]
  (junction 14) -> (junction 128) [order 1] : [tfv_va || tfv_vb || tfv_vc || tfv_iphasea || tfv_iphaseb || tfv_iphasec || tfv_vbulk || tfv_vmid /*|| tfv_vtop*/ || tfv_vaux || tz_ocp || tz_ovp || fault]
      | {
      | fault = true;
      | state = 1;
      | }
  (junction 542) -> (junction 501)
  (junction 501) -> (junction 544) [order 2]
  (junction 501) -> (junction 490) [order 1] : [fut_en_req]
  (junction 544) -> (junction 504)
  (junction 490) -> (junction 492) [order 1] : [!fut_en]
  (junction 504) -> (junction 506) [order 1] : [fut_en]
  (junction 492) -> (junction 498) : {
      | configFutEn();
      | fut_en = true;
      | }
  (junction 490) -> (junction 494) [order 2]
  (junction 504) -> (junction 512) [order 2]
  (junction 506) -> (junction 508) : {
      | configFutDis();
      | fut_en = false;
      | }
  (junction 494) -> (junction 498)
  (junction 508) -> (junction 512)
  (junction 498) -> (junction 520) : {state = 2;}
  (junction 512) -> (junction 346)
  (junction 346) -> (junction 339) [order 1] : [vbulk > 1573] //350V
  (junction 346) -> (junction 557) [order 2]
  (junction 339) -> (junction 329) : {
      | control_en = true;
      | enDigCmpMode();
      | }
  (junction 557) -> (junction 560) [order 1] : [vbulk < 1124] //250V
  (junction 557) -> (junction 558) [order 2]
  (junction 560) -> (junction 559) : {control_en = false;}
  (junction 558) -> (junction 559)
  (junction 559) -> (junction 329)
  (junction 329) -> (junction 114) [order 1] : [control_en]
  (junction 114) -> (junction 266) [order 1] : [vbulk > 1978] //440V
  (junction 329) -> (junction 580) [order 2]
  (junction 114) -> (junction 263) [order 2]
  (junction 266) -> (junction 273) : {
      | eoss = false;
      | burst_en = true;
      | }
  (junction 263) -> (junction 264) [order 1] : [vbulk < 1798] //400V
  (junction 263) -> (junction 267) [order 2]
  (junction 264) -> (junction 270) : {burst_en = false;}
  (junction 267) -> (junction 270)
  (junction 270) -> (junction 273)
  (junction 273) -> (junction 276) [order 1] : [burst_en]
  (junction 273) -> (junction 254) [order 2]
  (junction 276) -> (junction 327) : {
      | disablePwm();
      | va_seq = uint8(0); //forced zero
      | vb_seq = uint8(0);
      | vc_seq = uint8(0);
      | pha_en = false;
      | phb_en = false;
      | phc_en = false;
      | state = 5;
      | }
  (junction 254) -> (junction 256) [order 1] : [eoss]
  (junction 254) -> (junction 97) [order 2]
  (junction 256) -> (junction 101)
  (junction 580) -> (junction 581) [commented out] : [(grid_config_req != grid_config) || (singleph_config_req != singleph_config)]
  (junction 97) -> (junction 93) [order 1] : [(single(1798)-vbulk) > single(50)] //11V ripple
  (junction 580) -> (junction 583)
  (junction 581) -> (junction 582) [commented out] : {
      | configGrid(grid_config,   singleph_config);
      | grid_config = grid_config_req;
      | singleph_config = singleph_config_req;
      | }
  (junction 97) -> (junction 110) [order 2]
  (junction 93) -> (junction 109) : {ref = vbulk + single(50);
      | eoss = false;}
  (junction 110) -> (junction 96) [order 1] : [(single(1798)-vbulk) < single(-50)]
  (junction 110) -> (junction 94) [order 2] : {ref = single(1798); //400V
      | eoss = true;}
  (junction 96) -> (junction 108) : {ref = vbulk - single(50);
      | eoss = false;}
  (junction 101) -> (junction 352) [order 1] : [pha_en]
  (junction 109) -> (junction 101)
  (junction 582) -> (junction 583) [commented out]
  (junction 94) -> (junction 108)
  (junction 108) -> (junction 109)
  (junction 101) -> (junction 356) [order 2] : {
      | va_seq = uint8(0);
      | pha_en = detectZCPhA(van);
      | }
  (junction 352) -> (junction 354) : {va_seq = updateSequencePhA(van, ia);}
  (junction 583) -> (junction 133)
  (junction 356) -> (junction 354)
  (junction 354) -> (junction 362) [order 1] : [phb_en]
  (junction 354) -> (junction 365) [order 2] : {
      | vb_seq = uint8(0);
      | phb_en = detectZCPhB(vbn);
      | }
  (junction 362) -> (junction 366) : {vb_seq = updateSequencePhB(vbn, ib);}
  (junction 365) -> (junction 366)
  (junction 366) -> (junction 367) [order 1] : [phc_en]
  (junction 366) -> (junction 370) [order 2] : {
      | vc_seq = uint8(0);
      | phc_en = detectZCPhC(vcn);
      | }
  (junction 367) -> (junction 372) : {vc_seq = updateSequencePhC(vcn, ic);}
  (junction 370) -> (junction 372)
  (junction 372) -> (junction 299) : {state = 4;}
  (junction 128) -> (junction 133) : //{calib_ok = false;} //calib_ok resets at fault or CAN command
  (junction 133) -> (junction 299) : {
      | disablePwm();
      | control_en = false;
      | eoss = false;
      | disDigCmpMode();
      | pha_en = false;
      | phb_en = false;
      | phc_en = false;
      | ref = vbulk;
      | state = 3;
      | }
  (junction 299) -> (junction 327)
  (junction 327) -> (junction 533)
  (junction 539) -> (junction 520)
  (junction 520) -> (junction 533)
  data: grid_config function_input double size=1; sinlgeph_config function_input double size=1; van function_input double size=1; vbn function_input double size=1; vcn function_input double size=1; theta function_output double size=1; calib_ok function_output; cnt_calib function_input uint16 size=1; van function_input single size=1; vbn function_input single size=1; vcn function_input single size=1; ia function_input single size=1; ib function_input single size=1; ic function_input single size=1; vxn function_input; phx_en function_output; vxn function_input; phx_en function_output; vxn function_input; phx_en function_output; vxn function_input; vx_seq function_output; ix function_input; vxn function_input; vx_seq function_output; ix function_input; vxn function_input; vx_seq function_output; ix function_input; state output uint16 =0; calib_ok output boolean =false; van input single; vbn input single; vcn input single; ia input single; ib input single; ic input single; tfv_vbulk data_store_memory; tfv_va data_store_memory; tfv_vmid data_store_memory; tfv_vb data_store_memory; tfv_vc data_store_memory; tfv_iphasea data_store_memory; tfv_iphaseb data_store_memory; tfv_iphasec data_store_memory; tfv_vtop data_store_memory; control_en output boolean =false; burst_en output boolean =false; eoss output boolean =false; ref output single =0; va_seq output uint8 =false; vb_seq output uint8 =false; vc_seq output uint8 =false; vbulk input single; fault local boolean =false; cnt_calib data_store_memory =0; theta data_store_memory =0; fut_en_req input uint8; fut_en local boolean =false; tfv_vaux data_store_memory; tz_ocp data_store_memory; tz_ovp data_store_memory; cnt_200ms local uint16 =0; pha_en output boolean =false; phb_en output boolean =false; phc_en output boolean =false; grid_config_req input uint8; singleph_config_req input uint8; grid_config local uint8 =0; singleph_config local uint8 =0
